simulink model "problem4"  (R2024b)
settings: Solver=VariableStepAuto  StartTime=0.0  StopTime=4000  RelTol=1e-3
model workspace (MAT data in the model file):
  P0 = Simulink.Parameter
  P0.Value = [100  0  0  0; 0  100  0  0; 0  0  100  0; 0  0  0  100]
  P0.Complexity = 'real'
  P0.Dimensions = [4 4]
  P0.DataType = 'auto'
  alpha = Simulink.Parameter
  alpha.Value = [0.0001847; 0.0001922]
  alpha.Complexity = 'real'
  alpha.Dimensions = [2 1]
  alpha.DataType = 'auto'
  beta = Simulink.Parameter
  beta.Value = [0.8869; -1.885]
  beta.Complexity = 'real'
  beta.Dimensions = [2 1]
  beta.DataType = 'auto'
  g = Simulink.Parameter
  g.Value = 1
  g.Complexity = 'real'
  g.Dimensions = [1 1]
  g.DataType = 'auto'
settings Model: Creator=djd14  LastModifiedBy=djd14

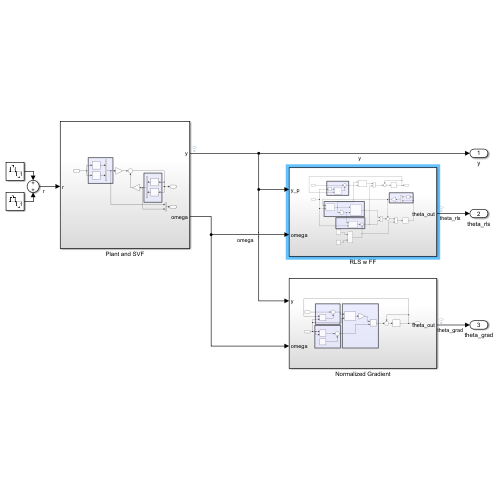
[thumbnail: Simulink's stored preview of the top-level diagram]
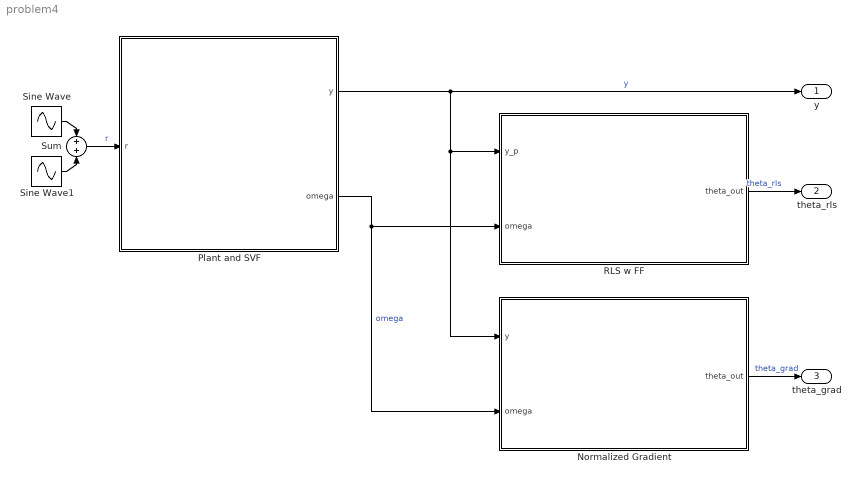
== system problem4 ==
  Normalized Gradient : Subsystem
  Plant and SVF : Subsystem
  RLS w FF : Subsystem
  Sine Wave : Sin  Frequency=0.02  SampleTime=1
  Sine Wave1 : Sin  SampleTime=1
  Sum : Sum  Inputs=+|+
  y : Outport  SampleTime=1
  theta_rls : Outport  Port=2
  theta_grad : Outport  Port=3
  wires:
  RLS w FF/1(theta_out) -> theta_rls/1  "theta_rls"
  Plant and SVF/2(omega) -> Normalized Gradient/2(omega), RLS w FF/2(omega)  "omega"
  Sine Wave1/1 -> Sum/2
  Sine Wave/1 -> Sum/1
  Plant and SVF/1(y) -> Normalized Gradient/1(y), RLS w FF/1(y_p), y/1  "y"
  Sum/1 -> Plant and SVF/1(r)  "r"
  Normalized Gradient/1(theta_out) -> theta_grad/1  "theta_grad"

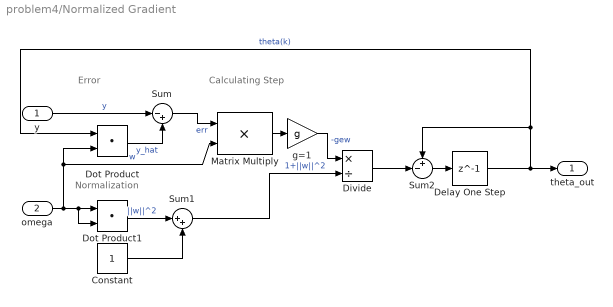
== system problem4/Normalized Gradient ==
  note: Calculating Step
  note: Normalization
  note: Error
  y : Inport
  omega : Inport  Port=2
  Constant : Constant
  Delay One Step : Delay  DelayLength=1
  Divide : Product  Inputs=*/
  Dot Product : DotProduct  OutDataTypeStr=Inherit: Inherit via internal rule
  Dot Product1 : DotProduct  OutDataTypeStr=Inherit: Inherit via internal rule
  Matrix Multiply : Product
  Sum : Sum  Inputs=|-+
  Sum1 : Sum  Inputs=|++
  Sum2 : Sum  Inputs=+-|
  g=1 : Gain  Gain=g
  theta_out : Outport
  wires:
  Dot Product/1 -> Sum/2  "y_hat"
  y/1 -> Sum/1  "y"
  omega/1 -> Dot Product1/1, Dot Product1/2, Matrix Multiply/2, Dot Product/2  "w"
  Delay One Step/1 -> Dot Product/1, Sum2/1, theta_out/1  "theta(k)"
  Dot Product1/1 -> Sum1/1  "||w||^2"
  Constant/1 -> Sum1/2
  Sum/1 -> Matrix Multiply/1  "err"
  Sum1/1 -> Divide/2  "1+||w||^2"
  Divide/1 -> Sum2/2
  Sum2/1 -> Delay One Step/1
  g=1/1 -> Divide/1  "-gew"
  Matrix Multiply/1 -> g=1/1

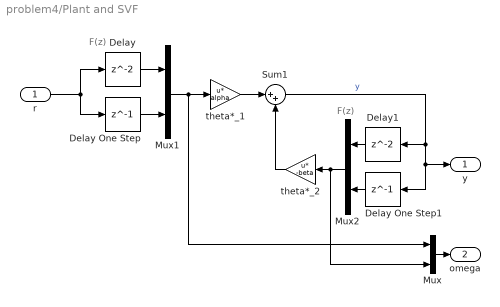
== system problem4/Plant and SVF ==
  note: F(z)
  note: F(z)
  r : Inport
  Delay : Delay
  Delay One Step : Delay  DelayLength=1
  Delay One Step1 : Delay  DelayLength=1
  Delay1 : Delay
  Mux : Mux  Inputs=2
  Mux1 : Mux  Inputs=2
  Mux2 : Mux  Inputs=2
  Sum1 : Sum  Inputs=|++
  theta*_1 : Gain  Gain=alpha  Multiplication=Matrix(u*K)
  theta*_2 : Gain  Gain=-beta  Multiplication=Matrix(u*K)
  y : Outport
  omega : Outport  Port=2
  wires:
  theta*_1/1 -> Sum1/1
  Mux2/1 -> Mux/2, theta*_2/1
  r/1 -> Delay One Step/1, Delay/1
  Sum1/1 -> Delay One Step1/1, y/1, Delay1/1  "y"
  Delay One Step/1 -> Mux1/2
  Delay One Step1/1 -> Mux2/2
  theta*_2/1 -> Sum1/2
  Delay/1 -> Mux1/1
  Delay1/1 -> Mux2/1
  Mux1/1 -> Mux/1, theta*_1/1
  Mux/1 -> omega/1

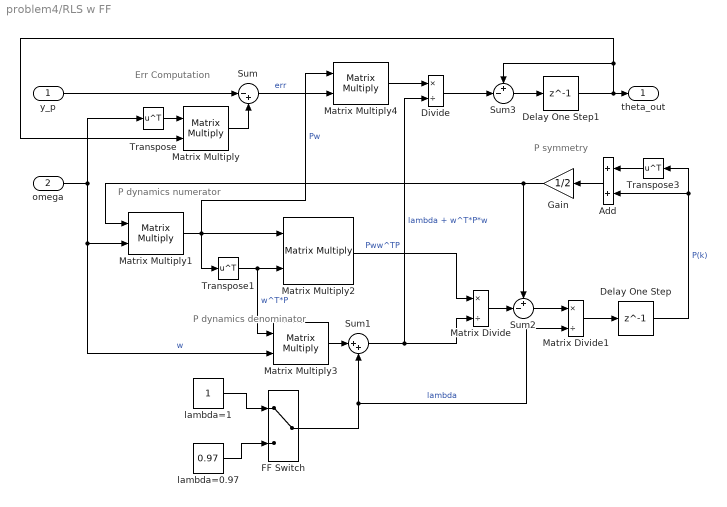
== system problem4/RLS w FF ==
  note: P symmetry
  note: P dynamics denominator
  note: P dynamics numerator
  note: Err Computation
  y_p : Inport
  omega : Inport  Port=2
  Add : Sum
  Delay One Step : Delay  DelayLength=1  InitialCondition=P0
  Delay One Step1 : Delay  DelayLength=1
  Divide : Product  Inputs=*/
  FF Switch : ManualSwitch
  Gain : Gain  Gain=1/2
  Matrix Divide : Product  Inputs=*/
  Matrix Divide1 : Product  Inputs=*/
  Matrix Multiply{,1..4} (5 alike) : Product  Multiplication=Matrix(*)
  Sum : Sum  Inputs=|-+
  Sum1 : Sum  Inputs=|++
  Sum2 : Sum  Inputs=+-|
  Sum3 : Sum  Inputs=+-|
  Transpose : Math  Operator=transpose
  Transpose1 : Math  Operator=transpose
  Transpose3 : Math  Operator=transpose
  lambda=0.97 : Constant  Value=0.97
  lambda=1 : Constant
  theta_out : Outport
  wires:
  omega/1 -> Transpose/1, Matrix Multiply3/2, Matrix Multiply1/2  "w"
  Transpose/1 -> Matrix Multiply/1
  y_p/1 -> Sum/1
  Matrix Multiply/1 -> Sum/2
  Sum/1 -> Matrix Multiply4/2  "err"
  Matrix Multiply1/1 -> Matrix Multiply4/1, Matrix Multiply2/1, Transpose1/1  "Pw"
  Delay One Step/1 -> Transpose3/1, Add/2  "P(k)"
  Matrix Multiply2/1 -> Matrix Divide/1  "Pww^TP"
  Transpose1/1 -> Matrix Multiply3/1, Matrix Multiply2/2  "w^T*P"
  Matrix Multiply3/1 -> Sum1/1
  Sum1/1 -> Divide/2, Matrix Divide/2  "lambda + w^T*P*w"
  Matrix Divide/1 -> Sum2/2
  Sum2/1 -> Matrix Divide1/1
  Matrix Divide1/1 -> Delay One Step/1
  Transpose3/1 -> Add/1
  Add/1 -> Gain/1
  Gain/1 -> Matrix Multiply1/1, Sum2/1
  FF Switch/1 -> Sum1/2, Matrix Divide1/2  "lambda"
  Sum3/1 -> Delay One Step1/1
  Delay One Step1/1 -> Sum3/1, Matrix Multiply/2, theta_out/1
  Matrix Multiply4/1 -> Divide/1
  Divide/1 -> Sum3/2
  lambda=1/1 -> FF Switch/1
  lambda=0.97/1 -> FF Switch/2
